simulink model "Bosch_VhclCtrl_AEB"  (R2021a)
settings: Solver=ode1  StartTime=0.0  StopTime=inf  FixedStep=0.001  RelTol=1e-3
PreLoadFcn:
  | vehicle = 'Car'; if ~length(which('cmself')), cmenv; end
  | Bosch_VhclCtrl_AEB_bus
InitFcn:
  | vehicle = 'Car'; if ~length(which('cmself')), cmenv; end
  | Bosch_VhclCtrl_AEB_bus
model workspace (MAT data in the model file):
  CritThreshold = 0.8
Description:
  | CarMaker Plug-in Model Target
settings Model: Creator=MAR3ABT  LastModifiedBy=MAR3ABT
settings RTWCC: Description=CarMaker Plug-in Model Target  SystemTargetFile=CarMaker.tlc  TemplateMakefile=CarMaker_unix-win64.tmf
settings CodeAppCC: MaxIdLength=127
settings STFCustomTargetCC: TargetLangStandard=C99 (ISO)  CombineOutputUpdateFcns=on  CodeInterfacePackaging=Reusable function  GRTInterface=off  GenerateAllocFcn=on  UseToolchainInfoCompliant=off  SystemTargetFile=CarMaker.tlc
settings GRTTargetCC: ParMdlRefBuildCompliant=off  CompOptLevelCompliant=off  ConcurrentExecutionCompliant=off  MatFileLogging=off  CodeInterfacePackaging=Reusable function  CPPClassGenCompliant=off  GenerateAllocFcn=on  UseToolchainInfoCompliant=off  RTWCAPIParams=on

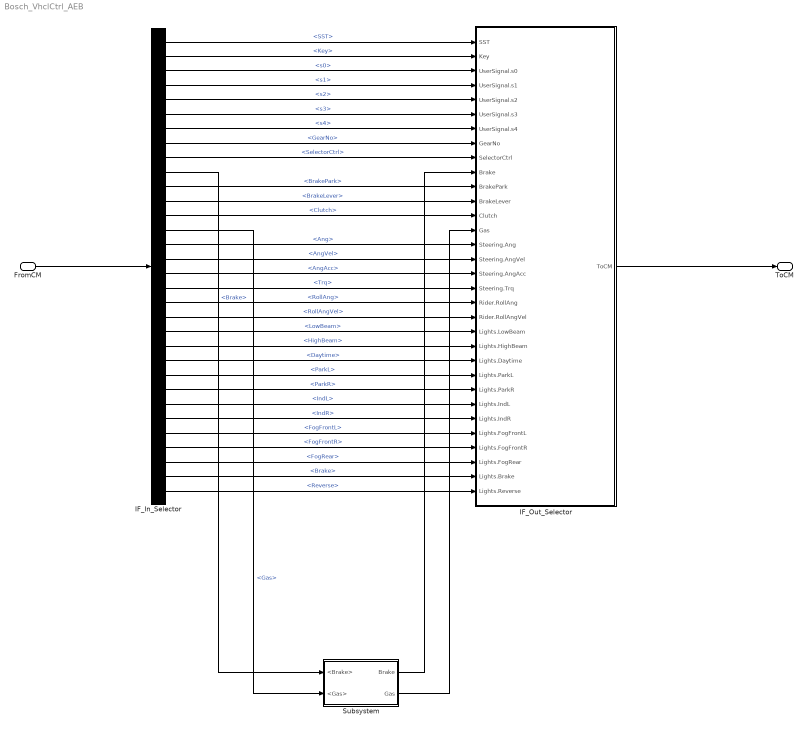
== system Bosch_VhclCtrl_AEB ==
  FromCM : Inport  OutDataTypeStr=Bus: cmVehicleControlIn
  IF_In_Selector : BusSelector  OutputSignals=SST,Key,UserSignal.s0,UserSignal.s1,UserSignal.s2,UserSignal.s3,UserSignal.s4,GearNo,SelectorCtrl,Brake,BrakePark,BrakeLever,Clutch,Gas,Steering.Ang,Steering.AngVel,Steering.AngAcc,Steering.Trq,Rider.RollAng,Rider.RollAngVel,Lights.LowBeam,Lights.HighBeam,Lights.Daytime,Lights.ParkL,Lights.ParkR,Lights.IndL,Lights.IndR,Lights.FogFrontL,Lights.FogFrontR,Lights.FogRear,Lights.Brake,Lights.Reverse
  IF_Out_Selector : Subsystem  mask(Signal Selection){}
      mask help: Signal Selection Block
      settings: OpenFcn=cmSignalSelect('SignalSelection_CB',gcb)
  Subsystem : Subsystem
  ToCM : Outport  OutDataTypeStr=Bus: cmVehicleControlOut
  wires:
  IF_In_Selector/3 -> IF_Out_Selector/3(UserSignal.s0)  "<s0>"
  IF_In_Selector/2 -> IF_Out_Selector/2(Key)  "<Key>"
  IF_In_Selector/4 -> IF_Out_Selector/4(UserSignal.s1)  "<s1>"
  IF_In_Selector/29 -> IF_Out_Selector/29(Lights.FogFrontR)  "<FogFrontR>"
  IF_In_Selector/19 -> IF_Out_Selector/19(Rider.RollAng)  "<RollAng>"
  IF_In_Selector/31 -> IF_Out_Selector/31(Lights.Brake)  "<Brake>"
  IF_In_Selector/14 -> Subsystem/2(<Gas>)  "<Gas>"
  IF_In_Selector/8 -> IF_Out_Selector/8(GearNo)  "<GearNo>"
  FromCM/1 -> IF_In_Selector/1
  IF_In_Selector/11 -> IF_Out_Selector/11(BrakePark)  "<BrakePark>"
  IF_In_Selector/12 -> IF_Out_Selector/12(BrakeLever)  "<BrakeLever>"
  IF_In_Selector/22 -> IF_Out_Selector/22(Lights.HighBeam)  "<HighBeam>"
  IF_In_Selector/21 -> IF_Out_Selector/21(Lights.LowBeam)  "<LowBeam>"
  IF_In_Selector/28 -> IF_Out_Selector/28(Lights.FogFrontL)  "<FogFrontL>"
  IF_In_Selector/17 -> IF_Out_Selector/17(Steering.AngAcc)  "<AngAcc>"
  IF_In_Selector/15 -> IF_Out_Selector/15(Steering.Ang)  "<Ang>"
  IF_In_Selector/27 -> IF_Out_Selector/27(Lights.IndR)  "<IndR>"
  IF_In_Selector/24 -> IF_Out_Selector/24(Lights.ParkL)  "<ParkL>"
  IF_In_Selector/13 -> IF_Out_Selector/13(Clutch)  "<Clutch>"
  IF_In_Selector/5 -> IF_Out_Selector/5(UserSignal.s2)  "<s2>"
  IF_In_Selector/7 -> IF_Out_Selector/7(UserSignal.s4)  "<s4>"
  IF_In_Selector/20 -> IF_Out_Selector/20(Rider.RollAngVel)  "<RollAngVel>"
  IF_In_Selector/9 -> IF_Out_Selector/9(SelectorCtrl)  "<SelectorCtrl>"
  IF_In_Selector/6 -> IF_Out_Selector/6(UserSignal.s3)  "<s3>"
  IF_In_Selector/10 -> Subsystem/1(<Brake>)  "<Brake>"
  Subsystem/1(Brake) -> IF_Out_Selector/10(Brake)
  IF_Out_Selector/1(ToCM) -> ToCM/1
  IF_In_Selector/23 -> IF_Out_Selector/23(Lights.Daytime)  "<Daytime>"
  IF_In_Selector/30 -> IF_Out_Selector/30(Lights.FogRear)  "<FogRear>"
  IF_In_Selector/18 -> IF_Out_Selector/18(Steering.Trq)  "<Trq>"
  IF_In_Selector/26 -> IF_Out_Selector/26(Lights.IndL)  "<IndL>"
  IF_In_Selector/25 -> IF_Out_Selector/25(Lights.ParkR)  "<ParkR>"
  IF_In_Selector/16 -> IF_Out_Selector/16(Steering.AngVel)  "<AngVel>"
  IF_In_Selector/32 -> IF_Out_Selector/32(Lights.Reverse)  "<Reverse>"
  IF_In_Selector/1 -> IF_Out_Selector/1(SST)  "<SST>"
  Subsystem/2(Gas) -> IF_Out_Selector/14(Gas)

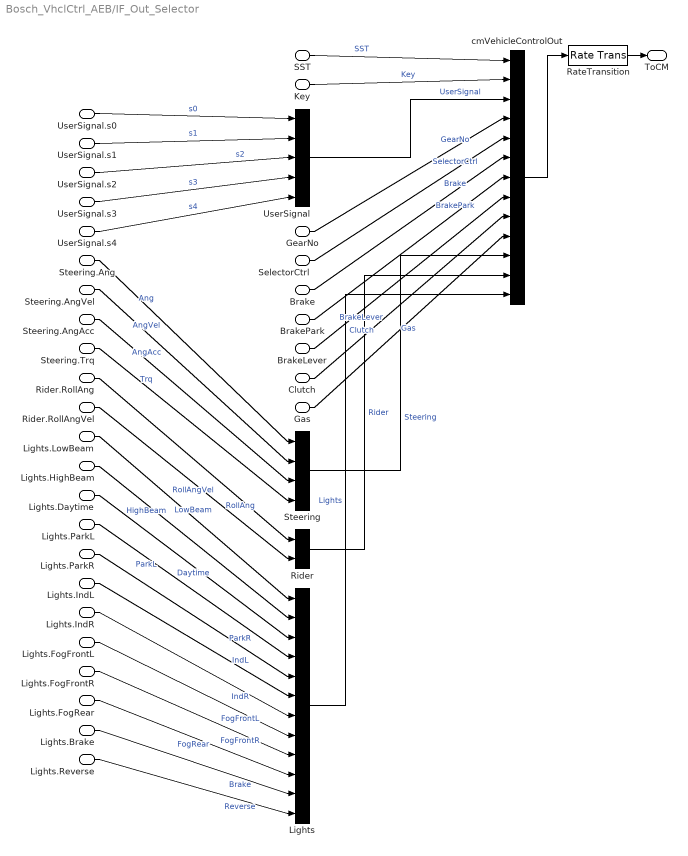
== system Bosch_VhclCtrl_AEB/IF_Out_Selector ==
  SST : Inport
  Key : Inport  Port=2
  UserSignal.s0 : Inport  Port=3
  UserSignal.s1 : Inport  Port=4
  UserSignal.s2 : Inport  Port=5
  UserSignal.s3 : Inport  Port=6
  UserSignal.s4 : Inport  Port=7
  GearNo : Inport  Port=8
  SelectorCtrl : Inport  Port=9
  Brake : Inport  Port=10
  BrakePark : Inport  Port=11
  BrakeLever : Inport  Port=12
  Clutch : Inport  Port=13
  Gas : Inport  Port=14
  Steering.Ang : Inport  Port=15
  Steering.AngVel : Inport  Port=16
  Steering.AngAcc : Inport  Port=17
  Steering.Trq : Inport  Port=18
  Rider.RollAng : Inport  Port=19
  Rider.RollAngVel : Inport  Port=20
  Lights.LowBeam : Inport  Port=21
  Lights.HighBeam : Inport  Port=22
  Lights.Daytime : Inport  Port=23
  Lights.ParkL : Inport  Port=24
  Lights.ParkR : Inport  Port=25
  Lights.IndL : Inport  Port=26
  Lights.IndR : Inport  Port=27
  Lights.FogFrontL : Inport  Port=28
  Lights.FogFrontR : Inport  Port=29
  Lights.FogRear : Inport  Port=30
  Lights.Brake : Inport  Port=31
  Lights.Reverse : Inport  Port=32
  Lights : BusCreator  Inputs=12
  RateTransition : RateTransition  OutPortSampleTime=str2num(get_param(bdroot,'FixedStep'))
  Rider : BusCreator  Inputs=2
  Steering : BusCreator  Inputs=4
  UserSignal : BusCreator  Inputs=5
  cmVehicleControlOut : BusCreator  Inputs=13
  ToCM : Outport
  wires:
  RateTransition/1 -> ToCM/1
  cmVehicleControlOut/1 -> RateTransition/1
  UserSignal/1 -> cmVehicleControlOut/3  "UserSignal"
  Steering/1 -> cmVehicleControlOut/11  "Steering"
  Rider/1 -> cmVehicleControlOut/12  "Rider"
  Lights/1 -> cmVehicleControlOut/13  "Lights"
  Brake/1 -> cmVehicleControlOut/6  "Brake"
  SST/1 -> cmVehicleControlOut/1  "SST"
  Key/1 -> cmVehicleControlOut/2  "Key"
  UserSignal.s0/1 -> UserSignal/1  "s0"
  UserSignal.s1/1 -> UserSignal/2  "s1"
  UserSignal.s2/1 -> UserSignal/3  "s2"
  UserSignal.s3/1 -> UserSignal/4  "s3"
  UserSignal.s4/1 -> UserSignal/5  "s4"
  GearNo/1 -> cmVehicleControlOut/4  "GearNo"
  SelectorCtrl/1 -> cmVehicleControlOut/5  "SelectorCtrl"
  BrakePark/1 -> cmVehicleControlOut/7  "BrakePark"
  BrakeLever/1 -> cmVehicleControlOut/8  "BrakeLever"
  Clutch/1 -> cmVehicleControlOut/9  "Clutch"
  Gas/1 -> cmVehicleControlOut/10  "Gas"
  Steering.Ang/1 -> Steering/1  "Ang"
  Steering.AngVel/1 -> Steering/2  "AngVel"
  Steering.AngAcc/1 -> Steering/3  "AngAcc"
  Steering.Trq/1 -> Steering/4  "Trq"
  Rider.RollAng/1 -> Rider/1  "RollAng"
  Rider.RollAngVel/1 -> Rider/2  "RollAngVel"
  Lights.LowBeam/1 -> Lights/1  "LowBeam"
  Lights.HighBeam/1 -> Lights/2  "HighBeam"
  Lights.Daytime/1 -> Lights/3  "Daytime"
  Lights.ParkL/1 -> Lights/4  "ParkL"
  Lights.ParkR/1 -> Lights/5  "ParkR"
  Lights.IndL/1 -> Lights/6  "IndL"
  Lights.IndR/1 -> Lights/7  "IndR"
  Lights.FogFrontL/1 -> Lights/8  "FogFrontL"
  Lights.FogFrontR/1 -> Lights/9  "FogFrontR"
  Lights.FogRear/1 -> Lights/10  "FogRear"
  Lights.Brake/1 -> Lights/11  "Brake"
  Lights.Reverse/1 -> Lights/12  "Reverse"

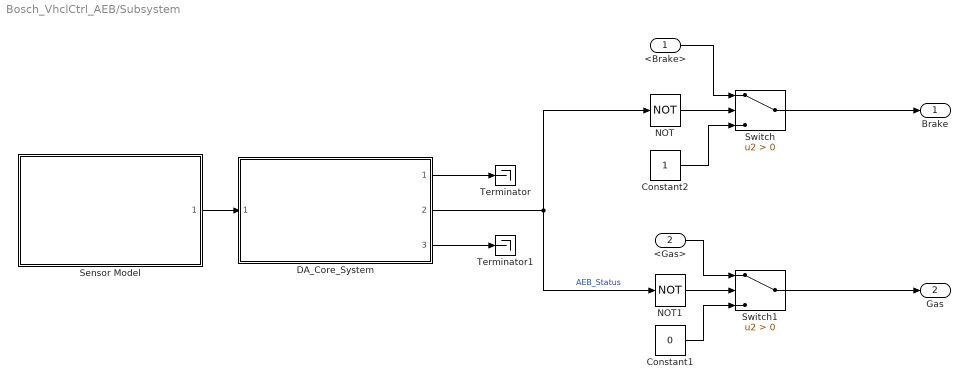
== system Bosch_VhclCtrl_AEB/Subsystem ==
  <Brake> : Inport
  <Gas> : Inport  Port=2
  Constant1 : Constant  Value=0
  Constant2 : Constant
  DA_Core_System : Subsystem  ReferencedSubsystem=DA_CoreSystem
  NOT : Logic  Operator=NOT  IconShape=distinctive  AllPortsSameDT=off  OutDataTypeStr=boolean
  NOT1 : Logic  Operator=NOT  IconShape=distinctive  AllPortsSameDT=off  OutDataTypeStr=boolean
  Sensor Model : Subsystem  ReferencedSubsystem=Sensor_Model_3V_1O
  Switch : Switch  Criteria=u2 > Threshold  OutDataTypeStr=Inherit: Same as first input
  Switch1 : Switch  Criteria=u2 > Threshold
  Terminator : Terminator
  Terminator1 : Terminator
  Brake : Outport
  Gas : Outport  Port=2
  wires:
  Constant1/1 -> Switch1/3
  Switch/1 -> Brake/1
  NOT/1 -> Switch/2
  <Gas>/1 -> Switch1/1
  Switch1/1 -> Gas/1
  <Brake>/1 -> Switch/1
  Constant2/1 -> Switch/3
  NOT1/1 -> Switch1/2
  DA_Core_System/2 -> NOT/1, NOT1/1  "AEB_Status"
  Sensor Model/1 -> DA_Core_System/1
  DA_Core_System/1 -> Terminator/1
  DA_Core_System/3 -> Terminator1/1
